simulink model "ManufacturingFacility"  (R2018b)
settings: Solver=VariableStepAuto  StartTime=0.0  StopTime=4000  RelTol=1e-3
undefined symbols (not defined in the file): m, n
settings Model: Creator=Ryan  LastModifiedBy=Ryan

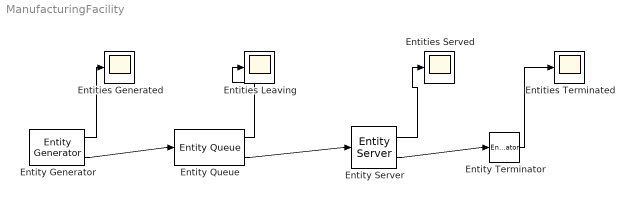
== system ManufacturingFacility ==
  Entities Generated : Scope
  Entities Leaving : Scope
  Entities Served : Scope
  Entities Terminated : Scope
  Entity Generator : EntityGenerator  OutputPortMessageModes=n,m  NumberEntitiesDeparted=on  EntityType=Structured  EntityTypeName=Entity
      settings: OutputPortMap=o0,o3
  Entity Queue : EntityQueue  InputPortMessageModes=m  OutputPortMessageModes=n,m  NumberEntitiesDeparted=on
      settings: OutputPortMap=o0,o5
  Entity Server : EntityServer  InputPortMessageModes=m  OutputPortMessageModes=n,m  Capacity=1  ServiceTimeSource=MATLAB action  ServiceTimeAction=dt = wblrnd(13,1);  NumberEntitiesDeparted=on
      settings: OutputPortMap=o0,o9
  Entity Terminator : EntityTerminator  InputPortMessageModes=m  NumberEntitiesArrived=on
      settings: OutputPortMap=o0
  wires:
  Entity Terminator/1 -> Entities Terminated/1
  Entity Queue/1 -> Entities Leaving/1
  Entity Generator/1 -> Entities Generated/1
  Entity Generator/2 -> Entity Queue/1
  Entity Queue/2 -> Entity Server/1
  Entity Server/2 -> Entity Terminator/1
  Entity Server/1 -> Entities Served/1
